simulink model "ranqilunji"  (R2014a)
settings: Solver=ode45  StartTime=0.0  StopTime=10.0  RelTol=1e-3
settings Model: Creator=Administrator  LastModifiedBy=Administrator

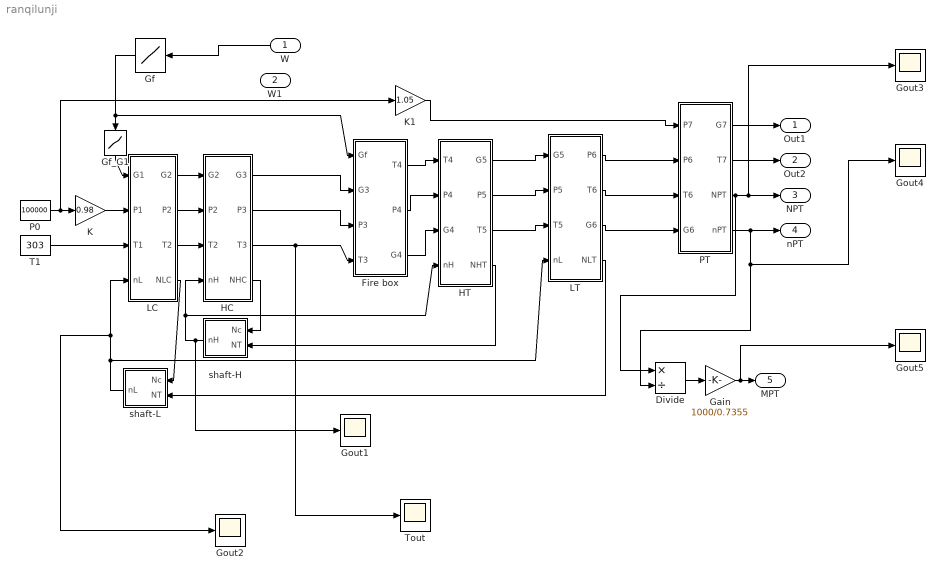
== system ranqilunji ==
  W : Inport
  W1 : Inport  Port=2
  Divide : Product  Inputs=*/
  Fire box : Subsystem
  Gain : Gain  Gain=1000/0.7355
  Gf : Lookup  InputValues=[0,0.03,0.07,0.09,0.11,0.13,0.17,0.2,0.23,0.26,0.28,0.3,0.32,0.34,0.35,0.38,0.4,0.42,0.44,0.47,0.49,0.5,0.52,0.54,0.55,0.59,0.61,0.64,0.66,0.68,0.7,0.72,0.74,0.77,0.81,0.83,0.85,0.88,0.93,0.95,0.97,1]  Table=[0.172,0.236,0.331,0.331,0.366,0.411,0.488,0.536,0.582,0.605,0.644,0.682,0.698,0.728,0.727,0.783,0.783,0.813,0.857,0.886,0.935,0.949,0.95,0.975,0.999,1.022,1.069,1.149,1.153,1.184,1.206,1.233,1.256,1.271,1.325,1.383,1.383,1.439,1.481,1.504,1.52,1.574]
  Gf_G1 : Lookup  InputValues=[0.172,0.236,0.331,0.366,0.411,0.488,0.536,0.582,0.605,0.644,0.682,0.698,0.727,0.728,0.783,0.813,0.857,0.886,0.935,0.949,0.95,0.975,0.999,1.022,1.069,1.149,1.153,1.184,1.206,1.233,1.256,1.271,1.325,1.383,1.439,1.481,1.504,1.52,1.574]  Table="[20.01, 25.93, 38.77,  43.65, 45.94, 51.85, 54.70, 56.85, 59.03, 61.91, 60.44, 61.58, 62.93, 63.04, 65.71,   67.00, 69.52, 70.63, 73.19, 73.46, 73.44, 73.83, 75.62, 76.39, 78.27, 81.17, 81.50, 82.44, 83.44, 84.31, 85.30, 86.17, 87.93, 89.72, 91.51, 93.65, 94.63, 94.92, 97.64]"
  Gout{1..5} (5 alike) : Scope
      Gout1 settings: TimeRange=10
      Gout2 settings: TimeRange=10  SaveName=ScopeData3
      Gout3 settings: TimeRange=10  SaveName=ScopeData21
      Gout4 settings: TimeRange=10  SaveName=ScopeData2
      Gout5 settings: TimeRange=10  SaveName=ScopeData5
  HC : Subsystem
  HT : Subsystem
  K : Gain  Gain=0.98
  K1 : Gain  Gain=1.05
  LC : Subsystem
  LT : Subsystem
  P0 : Constant  Value=100000
  PT : Subsystem
  T1 : Constant  Value=303
  Tout : Scope
      settings: TimeRange=200  YMin=740  YMax=790
  shaft-H : Subsystem  mask(rotor module){J=30}
      mask prompts: J "J moment of inertia(Nm)"
      mask help: (pi^2*J*n/900)*(dn/dt)=NT-Nc
  shaft-L : Subsystem  mask(rotor module){J=15}
      mask prompts: J "J moment of inertia(Nm)"
      mask help: (pi^2*J*n/900)*(dn/dt)=NT-Nc
  Out1 : Outport
  Out2 : Outport  Port=2
  NPT : Outport  Port=3
  nPT : Outport  Port=4
  MPT : Outport  Port=5
  wires:
  T1/1 -> LC/3(T1)
  K/1 -> LC/2(P1)
  LC/1(G2) -> HC/1(G2)
  LC/2(P2) -> HC/2(P2)
  LC/3(T2) -> HC/3(T2)
  HC/1(G3) -> Fire box/2(G3)
  HC/2(P3) -> Fire box/3(P3)
  HC/3(T3) -> Fire box/4(T3), Tout/1
  HC/4(NHC) -> shaft-H/1(Nc)
  HT/4(NHT) -> shaft-H/2(NT)
  shaft-H/1(nH) -> HT/4(nH), HC/4(nH), Gout1/1
  LC/4(NLC) -> shaft-L/1(Nc)
  LT/4(NLT) -> shaft-L/2(NT)
  Gf/1 -> Gf_G1/1, Fire box/1(Gf)
  Gf_G1/1 -> LC/1(G1)
  Fire box/3(G4) -> HT/3(G4)
  Fire box/2(P4) -> HT/2(P4)
  HT/3(T5) -> LT/3(T5)
  HT/2(P5) -> LT/2(P5)
  HT/1(G5) -> LT/1(G5)
  LT/3(G6) -> PT/4(G6)
  LT/2(T6) -> PT/3(T6)
  shaft-L/1(nL) -> LT/4(nL), LC/4(nL), Gout2/1
  LT/1(P6) -> PT/2(P6)
  P0/1 -> K/1, K1/1
  Fire box/1(T4) -> HT/1(T4)
  K1/1 -> PT/1(P7)
  W/1 -> Gf/1
  PT/1(G7) -> Out1/1
  PT/2(T7) -> Out2/1
  PT/3(NPT) -> Gout3/1, NPT/1, Divide/1
  PT/4(nPT) -> nPT/1, Gout4/1, Divide/2
  Gain/1 -> Gout5/1, MPT/1
  Divide/1 -> Gain/1

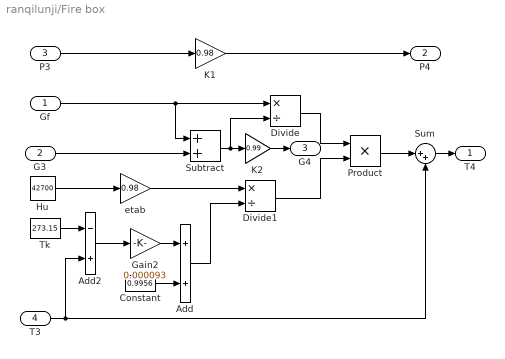
== system ranqilunji/Fire box ==
  Gf : Inport
  G3 : Inport  Port=2
  P3 : Inport  Port=3
  T3 : Inport  Port=4
  Add : Sum
  Add2 : Sum  Inputs=-+
  Constant : Constant  Value=0.9956
  Divide : Product  Inputs=*/
  Divide1 : Product  Inputs=*/
  Gain2 : Gain  Gain=0.000093
  Hu : Constant  Value=42700
  K1 : Gain  Gain=0.98
  K2 : Gain  Gain=0.99
  Product : Product  RndMeth=Zero
  Subtract : Sum
  Sum : Sum  Inputs=|++
  Tk : Constant  Value=273.15
  etab : Gain  Gain=0.98
  T4 : Outport
  P4 : Outport  Port=2
  G4 : Outport  Port=3
  wires:
  Gf/1 -> Divide/1, Subtract/1
  Divide/1 -> Product/1
  G3/1 -> Subtract/2
  Subtract/1 -> Divide/2, K2/1
  Hu/1 -> etab/1
  etab/1 -> Divide1/1
  Divide1/1 -> Product/2
  Product/1 -> Sum/1
  Sum/1 -> T4/1
  T3/1 -> Add2/2, Sum/2
  P3/1 -> K1/1
  K1/1 -> P4/1
  Constant/1 -> Add/2
  Gain2/1 -> Add/1
  Tk/1 -> Add2/1
  Add2/1 -> Gain2/1
  Add/1 -> Divide1/2
  K2/1 -> G4/1

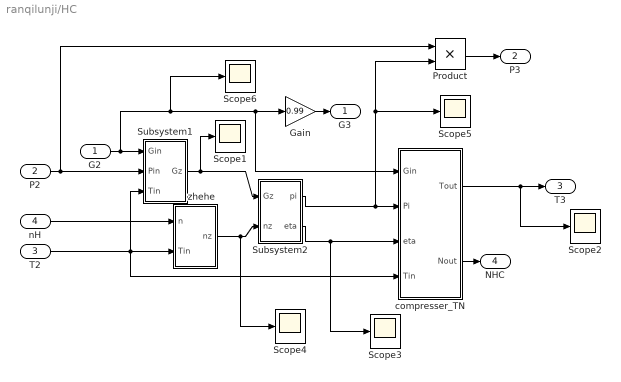
== system ranqilunji/HC ==
  G2 : Inport
  P2 : Inport  Port=2
  T2 : Inport  Port=3
  nH : Inport  Port=4
  Gain : Gain  Gain=0.99
  Product : Product  RndMeth=Zero
  Scope{1..6} (6 alike) : Scope
      Scope1 settings: YMin=2829.54  YMax=3127.38  SaveName=ScopeData16
      Scope2 settings: YMin=2829.54  YMax=3127.38  SaveName=ScopeData29
      Scope3 settings: YMin=2829.54  YMax=3127.38  SaveName=ScopeData24
      Scope4 settings: YMin=2829.54  YMax=3127.38  SaveName=ScopeData31
      Scope5 settings: YMin=2829.54  YMax=3127.38  SaveName=ScopeData10
      Scope6 settings: YMin=2829.54  YMax=3127.38  SaveName=ScopeData15
  Subsystem1 : Subsystem
  Subsystem2 : Subsystem
  compresser_TN : Subsystem  mask(Compressor_Tout Nout module){}
  zhehe : Subsystem
  G3 : Outport
  P3 : Outport  Port=2
  T3 : Outport  Port=3
  NHC : Outport  Port=4
  wires:
  zhehe/1(nz) -> Scope4/1, Subsystem2/2(nz)
  Subsystem2/1(pi) -> compresser_TN/2(Pi), Product/2, Scope5/1
  Subsystem2/2(eta) -> compresser_TN/3(eta), Scope3/1
  T2/1 -> zhehe/2(Tin), compresser_TN/4(Tin), Subsystem1/3(Tin)
  nH/1 -> zhehe/1(n)
  Gain/1 -> G3/1
  compresser_TN/1(Tout) -> T3/1, Scope2/1
  compresser_TN/2(Nout) -> NHC/1
  Subsystem1/1(Gz) -> Scope1/1, Subsystem2/1(Gz)
  G2/1 -> Subsystem1/1(Gin), Gain/1, compresser_TN/1(Gin), Scope6/1
  P2/1 -> Subsystem1/2(Pin), Product/1
  Product/1 -> P3/1

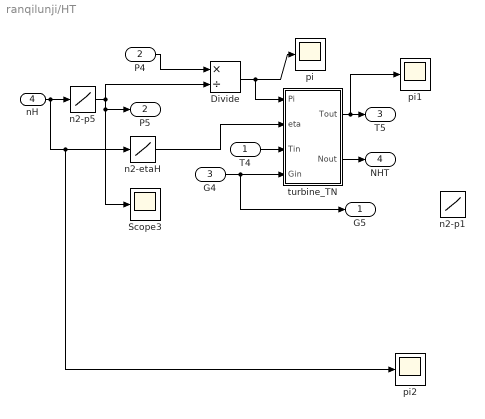
== system ranqilunji/HT ==
  T4 : Inport
  P4 : Inport  Port=2
  G4 : Inport  Port=3
  nH : Inport  Port=4
  Divide : Product  Inputs=*/
  Scope3 : Scope
      settings: TimeRange=100  YMin=5000  YMax=25000  SaveName=ScopeData34
  n2-etaH : Lookup  InputValues=[6000 6300 6500 6800 7000 7150 7300 7500 7800]  Table=[0.81 0.83 0.85 0.87 0.88 0.87 0.86 0.855 0.85]
  n2-p1 : Lookup  InputValues=[6000 6503 6995 7498 8002 8505 8997 9500]  Table=[139400 150700 186000 246700 332500 443400 575800 736100]
  n2-p5 : Lookup  InputValues=[5832,7212,7282,7644,7752,7853,8033,8092 8211 8392 8430 8452 8670 8767 8960 8999 9073]  Table=[154000,269000,296000,361000,391000,419000,476000,494000 534000 596000 609000 616000 684000 719000 806000 814000 831000]
  pi : Scope
      settings: TimeRange=100  YMin=2829.54  YMax=3127.38  SaveName=ScopeData17
  pi1 : Scope
      settings: TimeRange=100  YMin=2829.54  YMax=3127.38  SaveName=ScopeData7
  pi2 : Scope
      settings: TimeRange=100  YMin=2829.54  YMax=3127.38  SaveName=ScopeData35
  turbine_TN : Subsystem  mask(Turbine_Tout Nout module){}
  G5 : Outport
  P5 : Outport  Port=2
  T5 : Outport  Port=3
  NHT : Outport  Port=4
  wires:
  n2-etaH/1 -> turbine_TN/2(eta)
  P4/1 -> Divide/1
  nH/1 -> pi2/1, n2-etaH/1, n2-p5/1
  turbine_TN/1(Tout) -> T5/1, pi1/1
  T4/1 -> turbine_TN/3(Tin)
  turbine_TN/2(Nout) -> NHT/1
  G4/1 -> turbine_TN/4(Gin), G5/1
  Divide/1 -> turbine_TN/1(Pi), pi/1
  n2-p5/1 -> Divide/2, P5/1, Scope3/1

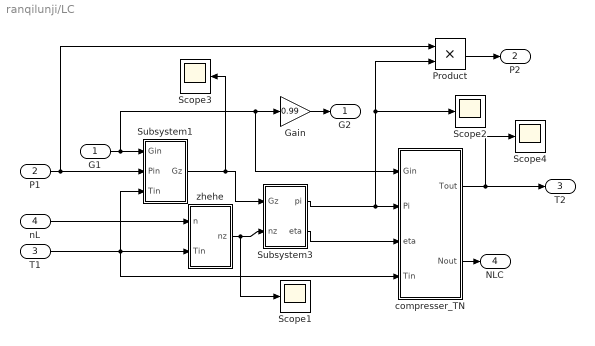
== system ranqilunji/LC ==
  G1 : Inport
  P1 : Inport  Port=2
  T1 : Inport  Port=3
  nL : Inport  Port=4
  Gain : Gain  Gain=0.99
  Product : Product  RndMeth=Zero
  Scope{1..4} (4 alike) : Scope
      Scope1 settings: YMin=2829.54  YMax=3127.38  SaveName=ScopeData14
      Scope2 settings: YMin=2829.54  YMax=3127.38  SaveName=ScopeData9
      Scope3 settings: YMin=2829.54  YMax=3127.38  SaveName=ScopeData30
      Scope4 settings: TimeRange=80  YMin=5000  YMax=30000  SaveName=ScopeData32
  Subsystem1 : Subsystem
  Subsystem3 : Subsystem
  compresser_TN : Subsystem  mask(Compressor_Tout Nout module){}
  zhehe : Subsystem
  G2 : Outport
  P2 : Outport  Port=2
  T2 : Outport  Port=3
  NLC : Outport  Port=4
  wires:
  zhehe/1(nz) -> Scope1/1, Subsystem3/2(nz)
  Subsystem3/1(pi) -> compresser_TN/2(Pi), Product/2, Scope2/1
  Subsystem3/2(eta) -> compresser_TN/3(eta)
  T1/1 -> zhehe/2(Tin), compresser_TN/4(Tin), Subsystem1/3(Tin)
  nL/1 -> zhehe/1(n)
  Gain/1 -> G2/1
  compresser_TN/1(Tout) -> T2/1, Scope4/1
  compresser_TN/2(Nout) -> NLC/1
  Subsystem1/1(Gz) -> Scope3/1, Subsystem3/1(Gz)
  G1/1 -> Subsystem1/1(Gin), Gain/1, compresser_TN/1(Gin)
  P1/1 -> Subsystem1/2(Pin), Product/1
  Product/1 -> P2/1

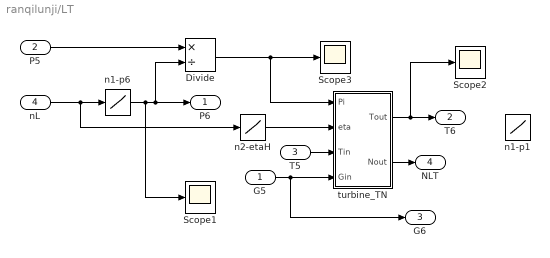
== system ranqilunji/LT ==
  G5 : Inport
  P5 : Inport  Port=2
  T5 : Inport  Port=3
  nL : Inport  Port=4
  Divide : Product  Inputs=*/
  Scope1 : Scope
      settings: TimeRange=100  YMin=5000  YMax=25000  SaveName=ScopeData28
  Scope2 : Scope
      settings: TimeRange=100  YMin=5000  YMax=25000  SaveName=ScopeData4
  Scope3 : Scope
      settings: TimeRange=100  YMin=5000  YMax=25000  SaveName=ScopeData20
  n1-p1 : Lookup  InputValues="[2849,4651,4850,5410,5586,5742,6024,6092,6102,6211,6385,6425 6435 6609 6698  6732 7015  7080 7185 ]"  Table="[101000,131000,141000,161000,171000,181000,201000,201000,211000,221000,241000,251000 251000 281000 291000  301000 321000  331000 341000]"
  n1-p6 : Lookup  InputValues=[2849,4651,4850,5410,5586,5742,6024,6092,6102,6211,6385,6425,6435,6609,6698,6732,7015,7080,7185]  Table=[113000,150000,157000,180000,190000,201000,221000,229000,229500,242000,267000,272000,277000,306000,321000,322000,354000,360000,371000]
  n2-etaH : Lookup  InputValues=[4300 5000 5500 6000 6500 7000 7500 8000 9000 9500]  Table=[0.82 0.83 0.835 0.84 0.85 0.86 0.875 0.87 0.865 0.86]
  turbine_TN : Subsystem  mask(Turbine_Tout Nout module){}
  P6 : Outport
  T6 : Outport  Port=2
  G6 : Outport  Port=3
  NLT : Outport  Port=4
  wires:
  n2-etaH/1 -> turbine_TN/2(eta)
  P5/1 -> Divide/1
  nL/1 -> n2-etaH/1, n1-p6/1
  turbine_TN/1(Tout) -> T6/1, Scope2/1
  T5/1 -> turbine_TN/3(Tin)
  turbine_TN/2(Nout) -> NLT/1
  G5/1 -> turbine_TN/4(Gin), G6/1
  n1-p6/1 -> Divide/2, P6/1, Scope1/1
  Divide/1 -> turbine_TN/1(Pi), Scope3/1

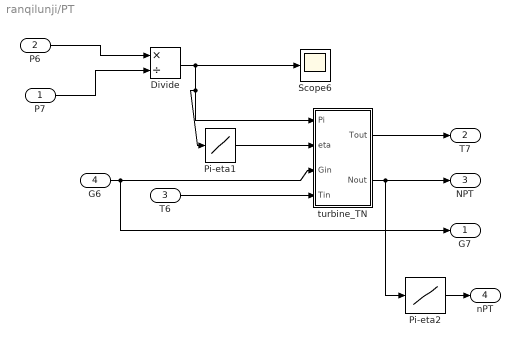
== system ranqilunji/PT ==
  P7 : Inport
  P6 : Inport  Port=2
  T6 : Inport  Port=3
  G6 : Inport  Port=4
  Divide : Product  Inputs=*/
  Pi-eta1 : Lookup  InputValues=[1,1.11 1.41 1.51 1.81 2.0 2.21 2.41 2.61 2.81]  Table=[0.825,0.83 0.85 0.86 0.88 0.90 0.905 0.91 0.905 0.9]
  Pi-eta2 : Lookup  InputValues=[307,625,1634,2141,2611,3121,4030,4941,5687,6256,6755,7309,7716,8175,8374,9153,9719,10196,10702,11284,11832,12033,12512,13051,13298,14334,14778,15580,16003,16531,16669,17381,17948,18600,19648,20212,20613,21462,22525,23139,23520,24372]  Table=[878,1243,1778,1749,1547,1574,1765,1930,2049,2045,2069,2150,2158,2185,2214,2272,2274,2209,2231,2240,2252,2500,2569,2649,2574,2650,2617,2639,2697,2653,2702,2785,2901,2979,3042,2919,2951,3108,3089,3056,3065,3142]
  Scope6 : Scope
      settings: YMin=2829.54  YMax=3127.38  SaveName=ScopeData22
  turbine_TN : Subsystem  mask(Turbine_Tout Nout module){}
  G7 : Outport
  T7 : Outport  Port=2
  NPT : Outport  Port=3
  nPT : Outport  Port=4
  wires:
  turbine_TN/1(Tout) -> T7/1
  turbine_TN/2(Nout) -> NPT/1, Pi-eta2/1
  G6/1 -> turbine_TN/3(Gin), G7/1
  Divide/1 -> Scope6/1, turbine_TN/1(Pi), Pi-eta1/1
  T6/1 -> turbine_TN/4(Tin)
  Pi-eta1/1 -> turbine_TN/2(eta)
  P6/1 -> Divide/1
  P7/1 -> Divide/2
  Pi-eta2/1 -> nPT/1

== system ranqilunji/shaft-H ==
  Nc : Inport
  NT : Inport  Port=2
  Add : Sum  Inputs=-+
  Divide : Product  Inputs=3
  Fcn : Fcn  Expr=1/u
  Fcn1 : Fcn  Expr=1/u
  Gain : Gain  Gain=15/(pi*pi)
  Gain3 : Gain  Gain=60
  Integrator : Integrator  InitialCondition=143.58
  J : Constant  Value=J
  nH : Outport
  wires:
  Nc/1 -> Add/1
  NT/1 -> Add/2
  Divide/1 -> Integrator/1
  Integrator/1 -> Fcn1/1, Gain3/1
  Add/1 -> Divide/1
  J/1 -> Fcn/1
  Gain/1 -> Divide/2
  Fcn/1 -> Gain/1
  Fcn1/1 -> Divide/3
  Gain3/1 -> nH/1

== system ranqilunji/shaft-L ==
  Nc : Inport
  NT : Inport  Port=2
  Add : Sum  Inputs=-+
  Divide : Product  Inputs=3
  Fcn : Fcn  Expr=1/u
  Fcn1 : Fcn  Expr=1/u
  Gain : Gain  Gain=15/(pi*pi)
  Gain2 : Gain  Gain=60
  Integrator : Integrator  InitialCondition=105.9
  J : Constant  Value=J
  nL : Outport
  wires:
  Nc/1 -> Add/1
  NT/1 -> Add/2
  Divide/1 -> Integrator/1
  Integrator/1 -> Fcn1/1, Gain2/1
  Add/1 -> Divide/1
  J/1 -> Fcn/1
  Gain/1 -> Divide/2
  Fcn/1 -> Gain/1
  Fcn1/1 -> Divide/3
  Gain2/1 -> nL/1

== system ranqilunji/HC/Subsystem1 ==
  Gin : Inport
  Pin : Inport  Port=2
  Tin : Inport  Port=3
  Divide : Product  Inputs=*/
  Divide1 : Product  Inputs=*/
  Divide2 : Product  Inputs=*/
  Fcn : Fcn  Expr=sqrt(u)
  P0 : Constant  Value=100000
  Product : Product  RndMeth=Zero
  T0 : Constant  Value=288
  Gz : Outport
  wires:
  Tin/1 -> Divide/1
  T0/1 -> Divide/2
  Divide/1 -> Fcn/1
  Pin/1 -> Divide1/1
  P0/1 -> Divide1/2
  Gin/1 -> Divide2/1
  Divide1/1 -> Divide2/2
  Fcn/1 -> Product/1
  Divide2/1 -> Product/2
  Product/1 -> Gz/1

== system ranqilunji/HC/Subsystem2 ==
  Gz : Inport
  nz : Inport  Port=2
  Lookup Table (2-D) : Lookup2D  RowIndex=[6000 6300 6500 6800 7000 7300 7500 7800]  ColumnIndex=[12:0.2:29]  Table=|
      | [2.4803 2.5510 2.6217 2.6924 2.7630 2.8337 2.9044 2.9751 3.0172 2.9863 2.9541 2.9206 2.8860 2.8500 2.8129 2.7745 2.7349 2.6940 2.6519 2.6085 2.5640 2.5181 2.4711 2.4906 2.5237 2.5573 2.5913 2.6257 2.6605 2.6958 2.7314 2.7675 2.8040 2.8409 2.8783 2.9161 2.9543 2.9929 3.0319 3.0714 3.1112 3.1515 3.1923 3.2334 3.2750 3.3169 3.3593 3.4022 3.4454 3.4891 3.5332 3.5777 3.6226 3.6679 3.7137 3.7599 3.8065 3.8535 3.9010 3.9488 3.9971 4.0307 4.0450 4.0645  4.0889 4.0613 4.0669 4.0759 4.0882 4.1107 4.1332 4.1561 4.2095 4.2632 4.3174 4.3720 4.4271 4.4825 4.5384 4.5947 4.6514 4.7085 4.7660 4.8240 4.8824 5.0412;
      | 2.4803 2.5510 2.6217 2.6924 2.7630 2.8337 2.9044 2.9751 3.0457 3.1164 3.1871 3.2578 3.3284 3.3991 3.5124 3.4922 3.4694 3.4440 3.4159 3.3853 3.3520 3.3161 3.2775 3.2364 3.1926 3.1462 3.0972 3.0456 2.9914 2.9345 2.8750 2.8129 2.8040 2.8409 2.8783 2.9161 2.9543 2.9929 3.0319 3.0714 3.1112 3.1515 3.1923 3.2334 3.2750 3.3169 3.3593 3.4022 3.4454 3.4891 3.5332 3.5777 3.6226 3.6679 3.7137 3.7599 3.8065 3.8535 3.9010 3.9488 3.9971 4.0307 4.0450 4.0645  4.0889 4.0613 4.0669 4.0759 4.0882 4.1107 4.1332 4.1561 4.2095 4.2632 4.3174 4.3720 4.4271 4.4825 4.5384 4.5947 4.6514 4.7085 4.7660 4.8240 4.8824 5.0412;
      | 2.4803 2.5510 2.6217 2.6924 2.7630 2.8337 2.9044 2.9751 3.0457 3.1164 3.1871 3.2578 3.3284 3.3991 3.4698 3.5405 3.6111 3.6818 3.7525 3.8394 3.8358 3.8266 3.8119 3.7916 3.7659 3.7345 3.6977 3.6553 3.6073 3.5539 3.4948 3.4303 3.3602 3.2845 3.2034 3.1167 3.0244 2.9929 3.0319 3.0714 3.1112 3.1515 3.1923 3.2334 3.2750 3.3169 3.3593 3.4022 3.4454 3.4891 3.5332 3.5777 3.6226 3.6679 3.7137 3.7599 3.8065 3.8535 3.9010 3.9488 3.9971 4.0307 4.0450 4.0645  4.0889 4.0613 4.0669 4.0759 4.0882 4.1107 4.1332 4.1561 4.2095 4.2632 4.3174 4.3720 4.4271 4.4825 4.5384 4.5947 4.6514 4.7085 4.7660 4.8240 4.8824 5.0412;
      | 2.4803 2.5510 2.6217 2.6924 2.7630 2.8337 2.9044 2.9751 3.0457 3.1164 3.1871 3.2578 3.3284 3.3991 3.4698 3.5405 3.6111 3.6818 3.7525 3.8231 3.8938 3.9645 4.0352 4.1058 4.1765 4.2472 4.3179 4.4049 4.4021 4.3892 4.3664 4.3334 4.2904 4.2374 4.1744 4.1012 4.0181 3.9249 3.8216 3.7083 3.5850 3.4516 3.3082 3.2334 3.2750 3.3169 3.3593 3.4022 3.4454 3.4891 3.5332 3.5777 3.6226 3.6679 3.7137 3.7599 3.8065 3.8535 3.9010 3.9488 3.9971 4.0307 4.0450 4.0645  4.0889 4.0613 4.0669 4.0759 4.0882 4.1107 4.1332 4.1561 4.2095 4.2632 4.3174 4.3720 4.4271 4.4825 4.5384 4.5947 4.6514 4.7085 4.7660 4.8240 4.8824 5.0412;
      | 2.4803 2.5510 2.6217 2.6924 2.7630 2.8337 2.9044 2.9751 3.0457 3.1164 3.1871 3.2578 3.3284 3.3991 3.4698 3.5405 3.6111 3.6818 3.7525 3.8231 3.8938 3.9645 4.0352 4.1058 4.1765 4.2472 4.3179 4.3885 4.4592 4.5299 4.6006 4.6379 4.6228 4.5996 4.5680 4.5283 4.4803 4.4241 4.3596 4.2869 4.2060 4.1168 4.0195 3.9138 3.8000 3.6779 3.5476 3.4090 3.4054 3.4591 3.5000 3.5277 3.5426 3.5679 3.5837 3.5999 3.8065 3.8535 3.9010 3.9488 3.9971 4.0307 4.0450 4.0645  4.0889 4.0613 4.0669 4.0759 4.0882 4.1107 4.1332 4.1561 4.2095 4.2632 4.3174 4.3720 4.4271 4.4825 4.5384 4.5947 4.6514 4.7085 4.7660 4.8240 4.8824 5.0412;
      | 2.4803 2.5510 2.6217 2.6924 2.7630 2.8337 2.9044 2.9751 3.0457 3.1164 3.1871 3.2578 3.3284 3.3991 3.4698 3.5405 3.6111 3.6818 3.7525 3.8231 3.8938 3.9645 4.0352 4.1058 4.1765 4.2472 4.3179 4.3885 4.4592 4.5299 4.6006 4.6712 4.7419 4.8126 4.8833 4.9539 5.0246 5.0953 5.1660 5.2000 5.1000 5.0000 4.9700 4.9000 4.8200 4.6810 4.6468 4.6015 4.5451 4.4775 4.3988 4.3090 4.2081 4.0961 3.9729 3.8386 3.8065 3.8535 3.9010 3.9488 3.9971 4.0307 4.0450 4.0645  4.0889 4.0613 4.0669 4.0759 4.0882 4.1107 4.1332 4.1561 4.2095 4.2632 4.3174 4.3720 4.4271 4.4825 4.5384 4.5947 4.6514 4.7085 4.7660 4.8240 4.8824 5.0412;
      | 2.4803 2.5510 2.6217 2.6924 2.7630 2.8337 2.9044 2.9751 3.0457 3.1164 3.1871 3.2578 3.3284 3.3991 3.4698 3.5405 3.6111 3.6818 3.7525 3.8231 3.8938 3.9645 4.0352 4.1058 4.1765 4.2472 4.3179 4.3885 4.4592 4.5299 4.6006 4.6712 4.7419 4.8126 4.8833 4.9539 5.0246 5.0953 5.1660 5.2366 5.3073 5.3780 5.4486 5.5193 5.5000 5.4500 5.4000 5.3500 5.3000 5.2500 5.2036 5.1763 5.1322 5.0715 4.9940 4.8998 4.7889 4.6613 4.5169 4.3559 4.0182 4.0307 4.0450 4.0645 4.0889 4.0613 4.0669 4.0759 4.0882 4.1107 4.1332 4.1561 4.2095 4.2632 4.3174 4.3720 4.4271 4.4825 4.5384 4.5947 4.6514 4.7085 4.7660 4.8240 4.8824 5.0412; 
      | 2.4803 2.5510 2.6217 2.6924 2.7630 2.8337 2.9044 2.9751 3.0457 3.1164 3.1871 3.2578 3.3284 3.3991 3.4698 3.5405 3.6111 3.6818 3.7525 3.8231 3.8938 3.9645 4.0352 4.1058 4.1765 4.2472 4.3179 4.3885 4.4592 4.5299 4.6006 4.6712 4.7419 4.8126 4.8833 4.9539 5.0246 5.0953 5.1660 5.2366 5.3073 5.3780 5.4486 5.5193 5.5900 5.6607 5.7313 5.8020 5.8727 5.9434 6.0140 6.0847 6.1554 6.2261 6.2967 6.3674 6.4381 6.5088 5.5861 5.3841 5.1514 4.8878 4.5936 4.0685 4.0889 4.0613 4.0669 4.0759 4.0882 4.1107 4.1332 4.1561 4.2095 4.2632 4.3174 4.3720 4.4271 4.4825 4.5384 4.5947 4.6514 4.7085 4.7660 4.8240 4.8824 5.0412;]
  Lookup Table (2-D)1 : Lookup2D  RowIndex=[6000 6300 6500 6800 7000 7300 7500 7800]  ColumnIndex=[12:0.2:29]  Table=|
      | [0.8450 0.8455 0.8460 0.8465 0.8470 0.8480 0.8490 0.8495 0.8500 0.8510 0.8520 0.8530 0.8540 0.8540 0.8540 0.8525 0.8510 0.8500 0.8490 0.8480 0.8470 0.8460 0.8450 0.8455 0.8460 0.8460 0.8460 0.8470 0.8480 0.8480 0.8480 0.8480 0.8480 0.8485 0.8490 0.8490 0.8490 0.8490 0.8490 0.8490 0.8490 0.8490 0.8490 0.8490 0.8490 0.8490 0.8490 0.8490 0.8490 0.8495 0.8500 0.8500 0.8500 0.8500 0.8500 0.8500 0.8500 0.8495 0.8490 0.8495 0.8500 0.8490 0.8480 0.8480 0.8480 0.8475 0.8470 0.8465 0.8460 0.8455 0.8450 0.8445 0.8440 0.8435 0.8430 0.8425 0.8420 0.8415 0.8410 0.8405 0.8400 0.8395 0.8390 0.8385 0.8380 0.8375;
      | 0.8450 0.8455 0.8460 0.8465 0.8470 0.8480 0.8490 0.8495 0.8500 0.8505 0.8510 0.8515 0.8520 0.8520 0.8520 0.8556 0.8597 0.8631 0.8658 0.8678 0.8691 0.8697 0.8696 0.8688 0.8672 0.8650 0.8621 0.8585 0.8542 0.8492 0.8435 0.8371 0.8480 0.8485 0.8490 0.8490 0.8490 0.8490 0.8490 0.8490 0.8490 0.8490 0.8490 0.8490 0.8490 0.8490 0.8490 0.8490 0.8490 0.8495 0.8500 0.8500 0.8500 0.8500 0.8500 0.8500 0.8500 0.8495 0.8490 0.8495 0.8500 0.8490 0.8480 0.8480 0.8480 0.8475 0.8470 0.8465 0.8460 0.8455 0.8450 0.8445 0.8440 0.8435 0.8430 0.8425 0.8420 0.8415 0.8410 0.8405 0.8400 0.8395 0.8390 0.8385 0.8380 0.8375;
      | 0.8450 0.8455 0.8460 0.8465 0.8470 0.8480 0.8490 0.8495 0.8500 0.8505 0.8510 0.8515 0.8520 0.8520 0.8520 0.8525 0.8530 0.8530 0.8530 0.8611 0.8688 0.8754 0.8809 0.8854 0.8888 0.8910 0.8922 0.8923 0.8914 0.8893 0.8861 0.8819 0.8766 0.8702 0.8627 0.8541 0.8444 0.8490 0.8490 0.8490 0.8490 0.8490 0.8490 0.8490 0.8490 0.8490 0.8490 0.8490 0.8490 0.8495 0.8500 0.8500 0.8500 0.8500 0.8500 0.8500 0.8500 0.8495 0.8490 0.8495 0.8500 0.8490 0.8480 0.8480 0.8480 0.8475 0.8470 0.8465 0.8460 0.8455 0.8450 0.8445 0.8440 0.8435 0.8430 0.8425 0.8420 0.8415 0.8410 0.8405 0.8400 0.8395 0.8390 0.8385 0.8380 0.8375;
      | 0.8450 0.8455 0.8460 0.8465 0.8470 0.8480 0.8490 0.8495 0.8500 0.8505 0.8510 0.8515 0.8520 0.8520 0.8520 0.8525 0.8530 0.8530 0.8530 0.8540 0.8550 0.8565 0.8580 0.8600 0.8620 0.8630 0.8640 0.8669 0.8710 0.8830 0.8930 0.9010 0.9070 0.9110 0.9129 0.9129 0.9108 0.9067 0.9006 0.8925 0.8824 0.8703 0.8561 0.8490 0.8490 0.8490 0.8490 0.8490 0.8490 0.8495 0.8500 0.8500 0.8500 0.8500 0.8500 0.8500 0.8500 0.8495 0.8490 0.8495 0.8500 0.8490 0.8480 0.8480 0.8480 0.8475 0.8470 0.8465 0.8460 0.8455 0.8450 0.8445 0.8440 0.8435 0.8430 0.8425 0.8420 0.8415 0.8410 0.8405 0.8400 0.8395 0.8390 0.8385 0.8380 0.8375;
      | 0.8450 0.8455 0.8460 0.8465 0.8470 0.8480 0.8490 0.8495 0.8500 0.8505 0.8510 0.8515 0.8520 0.8520 0.8520 0.8525 0.8530 0.8530 0.8530 0.8540 0.8550 0.8565 0.8580 0.8600 0.8620 0.8630 0.8640 0.8505 0.8500 0.8500 0.8500 0.8499 0.8618 0.8720 0.8808 0.8879 0.8935 0.8975 0.8999 0.9008 0.9001 0.8978 0.8940 0.8886 0.8816 0.8731 0.8630 0.8513 0.8490 0.8495 0.8500 0.8500 0.8500 0.8500 0.8500 0.8500 0.8500 0.8495 0.8490 0.8495 0.8500 0.8490 0.8480 0.8480 0.8480 0.8475 0.8470 0.8465 0.8460 0.8455 0.8450 0.8445 0.8440 0.8435 0.8430 0.8425 0.8420 0.8415 0.8410 0.8405 0.8400 0.8395 0.8390 0.8385 0.8380 0.8375;
      | 0.8450 0.8455 0.8460 0.8465 0.8470 0.8480 0.8490 0.8495 0.8500 0.8505 0.8510 0.8515 0.8520 0.8520 0.8520 0.8525 0.8530 0.8530 0.8530 0.8540 0.8550 0.8565 0.8580 0.8600 0.8620 0.8630 0.8640 0.8505 0.8500 0.8500 0.8500 0.8495 0.8490 0.8485 0.8480 0.8475 0.8470 0.8470 0.8470 0.8586 0.8661 0.8726 0.8781 0.8825 0.8860 0.8884 0.8897 0.8901 0.8894 0.8878 0.8851 0.8813 0.8766 0.8708 0.8640 0.8562 0.8500 0.8495 0.8490 0.8495 0.8500 0.8490 0.8480 0.8480 0.8480 0.8475 0.8470 0.8465 0.8460 0.8455 0.8450 0.8445 0.8440 0.8435 0.8430 0.8425 0.8420 0.8415 0.8410 0.8405 0.8400 0.8395 0.8390 0.8385 0.8380 0.8375;
      | 0.8450 0.8455 0.8460 0.8465 0.8470 0.8480 0.8490 0.8495 0.8500 0.8505 0.8510 0.8515 0.8520 0.8520 0.8520 0.8525 0.8530 0.8530 0.8530 0.8540 0.8550 0.8565 0.8580 0.8600 0.8620 0.8630 0.8640 0.8505 0.8500 0.8500 0.8500 0.8495 0.8490 0.8485 0.8480 0.8475 0.8470 0.8470 0.8470 0.8465 0.8460 0.8455 0.8450 0.8450 0.8450 0.8460 0.8456 0.8496 0.8528 0.8554 0.8572 0.8582 0.8585 0.8581 0.8569 0.8550 0.8523 0.8500 0.8500 0.8495 0.8495 0.8490 0.8480 0.8480 0.8480 0.8475 0.8470 0.8465 0.8460 0.8455 0.8450 0.8445 0.8440 0.8435 0.8430 0.8425 0.8420 0.8415 0.8410 0.8405 0.8400 0.8395 0.8390 0.8385 0.8380 0.8375;
      | 0.8450 0.8455 0.8460 0.8465 0.8470 0.8480 0.8490 0.8495 0.8500 0.8505 0.8510 0.8515 0.8520 0.8520 0.8520 0.8525 0.8530 0.8530 0.8530 0.8540 0.8550 0.8565 0.8580 0.8600 0.8620 0.8630 0.8640 0.8505 0.8500 0.8500 0.8500 0.8495 0.8490 0.8485 0.8480 0.8475 0.8470 0.8470 0.8470 0.8465 0.8460 0.8455 0.8450 0.8450 0.8450 0.8445 0.8440 0.8445 0.8450 0.8445 0.8440 0.8425 0.8400 0.8415 0.8430 0.8455 0.8480 0.8510 0.8550 0.8600 0.8650 0.8650 0.8650 0.8650 0.8480 0.8475 0.8470 0.8465 0.8460 0.8455 0.8450 0.8445 0.8440 0.8435 0.8430 0.8425 0.8420 0.8415 0.8410 0.8405 0.8400 0.8395 0.8390 0.8385 0.8380 0.8375;]
  pi : Outport
  eta : Outport  Port=2
  wires:
  nz/1 -> Lookup Table (2-D)/1, Lookup Table (2-D)1/1
  Gz/1 -> Lookup Table (2-D)1/2, Lookup Table (2-D)/2
  Lookup Table (2-D)/1 -> pi/1
  Lookup Table (2-D)1/1 -> eta/1

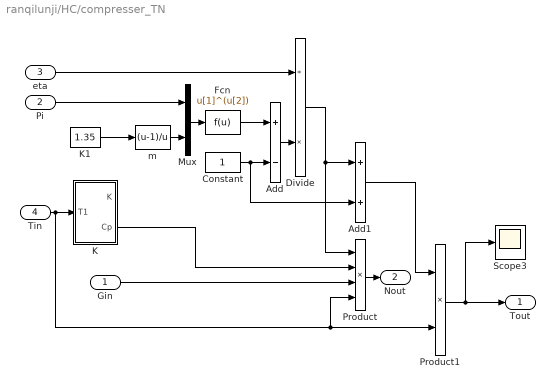
== system ranqilunji/HC/compresser_TN ==
  Gin : Inport
  Pi : Inport  Port=2
  eta : Inport  Port=3
  Tin : Inport  Port=4
  Add : Sum  Inputs=+-
  Add1 : Sum
  Constant : Constant
  Divide : Product  Inputs=/*
  Fcn : Fcn  Expr=u[1]^(u[2])
  K : Subsystem
  K1 : Constant  Value=1.35
  Mux : Mux  Inputs=2
  Product : Product  Inputs=4  RndMeth=Zero
  Product1 : Product  RndMeth=Zero
  Scope3 : Scope
      settings: YMin=2829.54  YMax=3127.38  SaveName=ScopeData18
  m : Fcn  Expr=(u-1)/u
  Tout : Outport
  Nout : Outport  Port=2
  wires:
  Tin/1 -> K/1(T1), Product1/2, Product/4
  Pi/1 -> Mux/1
  m/1 -> Mux/2
  Mux/1 -> Fcn/1
  Fcn/1 -> Add/1
  Add/1 -> Divide/2
  Divide/1 -> Add1/1, Product/1
  Constant/1 -> Add/2, Add1/2
  Product1/1 -> Tout/1, Scope3/1
  Product/1 -> Nout/1
  Add1/1 -> Product1/1
  K/2(Cp) -> Product/2
  Gin/1 -> Product/3
  eta/1 -> Divide/1
  K1/1 -> m/1

== system ranqilunji/HC/zhehe ==
  n : Inport
  Tin : Inport  Port=2
  Divide : Product  Inputs=*/
  Fcn : Fcn  Expr=sqrt(u/288)
  nz : Outport
  wires:
  Tin/1 -> Fcn/1
  n/1 -> Divide/1
  Fcn/1 -> Divide/2
  Divide/1 -> nz/1

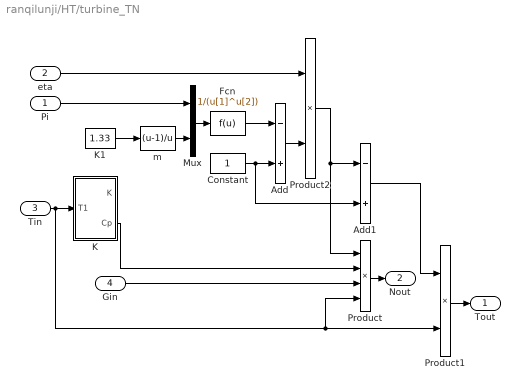
== system ranqilunji/HT/turbine_TN ==
  Pi : Inport
  eta : Inport  Port=2
  Tin : Inport  Port=3
  Gin : Inport  Port=4
  Add : Sum  Inputs=-+
  Add1 : Sum  Inputs=-+
  Constant : Constant
  Fcn : Fcn  Expr=1/(u[1]^u[2])
  K : Subsystem
  K1 : Constant  Value=1.33
  Mux : Mux  Inputs=2
  Product : Product  Inputs=4  RndMeth=Zero
  Product1 : Product  RndMeth=Zero
  Product2 : Product  RndMeth=Zero
  m : Fcn  Expr=(u-1)/u
  Tout : Outport
  Nout : Outport  Port=2
  wires:
  Tin/1 -> K/1(T1), Product1/2, Product/4
  Pi/1 -> Mux/1
  m/1 -> Mux/2
  Mux/1 -> Fcn/1
  Fcn/1 -> Add/1
  Add/1 -> Product2/2
  eta/1 -> Product2/1
  Product2/1 -> Add1/1, Product/1
  Constant/1 -> Add/2, Add1/2
  Product1/1 -> Tout/1
  Product/1 -> Nout/1
  Add1/1 -> Product1/1
  K/2(Cp) -> Product/2
  Gin/1 -> Product/3
  K1/1 -> m/1

== system ranqilunji/LC/Subsystem1 ==
  Gin : Inport
  Pin : Inport  Port=2
  Tin : Inport  Port=3
  Divide : Product  Inputs=*/
  Divide1 : Product  Inputs=*/
  Divide2 : Product  Inputs=*/
  Fcn : Fcn  Expr=sqrt(u)
  P0 : Constant  Value=100000
  Product : Product  RndMeth=Zero
  T0 : Constant  Value=288
  Gz : Outport
  wires:
  Tin/1 -> Divide/1
  T0/1 -> Divide/2
  Divide/1 -> Fcn/1
  Pin/1 -> Divide1/1
  P0/1 -> Divide1/2
  Gin/1 -> Divide2/1
  Divide1/1 -> Divide2/2
  Fcn/1 -> Product/1
  Divide2/1 -> Product/2
  Product/1 -> Gz/1

== system ranqilunji/LC/Subsystem3 ==
  Gz : Inport
  nz : Inport  Port=2
  Lookup Table (2-D) : Lookup2D  RowIndex=[4300 5000 5500 6000 6500 7000 7500 8000]  ColumnIndex=[20:0.5:100]  Table=|
      | [1.1111 1.1471 1.1832 1.2192 1.2552 1.2913 1.3273 1.3633 1.3994 1.4354 1.4714 1.5074 1.5435 1.5795 1.6155 1.6516 1.6876 1.7236 1.8750 1.8749 1.8720 1.8623 1.8457 1.8223 1.7920 1.7549 1.7109 1.6601 1.6024 1.5378 1.4664 1.3881 1.2420 1.2701 1.2983 1.3265 1.3547 1.3828 1.4110 1.4392 1.4673 1.4955 1.5237 1.5519 1.5800 1.6082 1.6364 1.6645 1.6927 1.7209 1.7491 1.7772 1.8054 1.8336 1.8617 1.8899 1.9181 1.9463 1.9744 2.0026 2.0308 2.0590 2.0871 2.1153 2.1435 2.1716 2.1998 2.2280 2.2562 2.2843 2.3125 2.3407 2.3688 2.3970 2.4252 2.4534 2.4815 2.5097 2.5379 2.5660 2.5942 2.6224 2.6506 2.6787 2.7069 2.7351 2.7633 2.7914 2.8196 2.8478 2.8759 2.9041 2.9323 2.9605 2.9886 3.0168 3.0450 3.0731 3.1013 3.1295 3.1577 3.1858 3.2140 3.2422 3.2703 3.2985 3.3267 3.3549 3.3830 3.4112 3.4394 3.4676 3.4957 3.5239 3.5521 3.5802 3.6084 3.6366 3.6648 3.6929 3.7211 3.7493 3.7774 3.8056 3.8338 3.8620 3.8901 3.9183 3.9465 3.9746 4.0028 4.0310 4.0592 4.0873 4.1155 4.1437 4.1719 4.2000 4.2282 4.2564 4.2845 4.3127 4.3409 4.3691 4.3972 4.4254 4.4536 4.4817 4.5099 4.5381 4.5663 4.5944 4.6226 4.6508 4.6789 4.7071 4.7353 4.7635 4.7916 4.8198 4.8480;
      | 1.1111 1.1471 1.1832 1.2192 1.2552 1.2913 1.3273 1.3633 1.3994 1.4354 1.4714 1.5074 1.5435 1.5795 1.6155 1.6516 1.6876 1.7236 1.7597 1.7957 1.8317 1.8678 1.9038 1.9398 1.9758 2.0119 2.0479 2.0839 2.1200 2.1560 2.1920 2.2281 2.2641 2.3001 2.3361 2.3722 2.4082 2.4442 2.4803 2.5163 2.5523 2.5884 2.5200 2.4780 2.3700 2.2800 2.1500 1.8820 1.6080 1.7209 1.7491 1.7772 1.8054 1.8336 1.8617 1.8899 1.9181 1.9463 1.9744 2.0026 2.0308 2.0590 2.0871 2.1153 2.1435 2.1716 2.1998 2.2280 2.2562 2.2843 2.3125 2.3407 2.3688 2.3970 2.4252 2.4534 2.4815 2.5097 2.5379 2.5660 2.5942 2.6224 2.6506 2.6787 2.7069 2.7351 2.7633 2.7914 2.8196 2.8478 2.8759 2.9041 2.9323 2.9605 2.9886 3.0168 3.0450 3.0731 3.1013 3.1295 3.1577 3.1858 3.2140 3.2422 3.2703 3.2985 3.3267 3.3549 3.3830 3.4112 3.4394 3.4676 3.4957 3.5239 3.5521 3.5802 3.6084 3.6366 3.6648 3.6929 3.7211 3.7493 3.7774 3.8056 3.8338 3.8620 3.8901 3.9183 3.9465 3.9746 4.0028 4.0310 4.0592 4.0873 4.1155 4.1437 4.1719 4.2000 4.2282 4.2564 4.2845 4.3127 4.3409 4.3691 4.3972 4.4254 4.4536 4.4817 4.5099 4.5381 4.5663 4.5944 4.6226 4.6508 4.6789 4.7071 4.7353 4.7635 4.7916 4.8198 4.8480;
      | 1.1111 1.1471 1.1832 1.2192 1.2552 1.2913 1.3273 1.3633 1.3994 1.4354 1.4714 1.5074 1.5435 1.5795 1.6155 1.6516 1.6876 1.7236 1.7597 1.7957 1.8317 1.8678 1.9038 1.9398 1.9758 2.0119 2.0479 2.0839 2.1200 2.1560 2.1920 2.2281 2.2641 2.3001 2.3361 2.3722 2.4082 2.4442 2.4803 2.5163 2.5523 2.5884 2.6244 2.6604 2.6965 2.7325 2.7685 2.8045 2.8406 2.8766 2.9126 2.9487 2.9847 3.0207 2.8905 2.8292 2.7444 2.6661 2.5443 2.4489 2.3700 2.1776 2.0217 2.1153 2.1435 2.1716 2.1998 2.2280 2.2562 2.2843 2.3125 2.3407 2.3688 2.3970 2.4252 2.4534 2.4815 2.5097 2.5379 2.5660 2.5942 2.6224 2.6506 2.6787 2.7069 2.7351 2.7633 2.7914 2.8196 2.8478 2.8759 2.9041 2.9323 2.9605 2.9886 3.0168 3.0450 3.0731 3.1013 3.1295 3.1577 3.1858 3.2140 3.2422 3.2703 3.2985 3.3267 3.3549 3.3830 3.4112 3.4394 3.4676 3.4957 3.5239 3.5521 3.5802 3.6084 3.6366 3.6648 3.6929 3.7211 3.7493 3.7774 3.8056 3.8338 3.8620 3.8901 3.9183 3.9465 3.9746 4.0028 4.0310 4.0592 4.0873 4.1155 4.1437 4.1719 4.2000 4.2282 4.2564 4.2845 4.3127 4.3409 4.3691 4.3972 4.4254 4.4536 4.4817 4.5099 4.5381 4.5663 4.5944 4.6226 4.6508 4.6789 4.7071 4.7353 4.7635 4.7916 4.8198 4.8480;
      | 1.1111 1.1471 1.1832 1.2192 1.2552 1.2913 1.3273 1.3633 1.3994 1.4354 1.4714 1.5074 1.5435 1.5795 1.6155 1.6516 1.6876 1.7236 1.7597 1.7957 1.8317 1.8678 1.9038 1.9398 1.9758 2.0119 2.0479 2.0839 2.1200 2.1560 2.1920 2.2281 2.2641 2.3001 2.3361 2.3722 2.4082 2.4442 2.4803 2.5163 2.5523 2.5884 2.6244 2.6604 2.6965 2.7325 2.7685 2.8045 2.8406 2.8766 2.9126 2.9487 2.9847 3.0207 3.0568 3.0928 3.1288 3.1648 3.2009 3.2369 3.2729 3.3090 3.3450 3.3810 3.3655 3.3396 3.3040 3.2587 3.2037 3.1389 3.0645 2.9803 2.8865 2.7829 2.6696 2.5466 2.4815 2.5097 2.5379 2.5660 2.5942 2.6224 2.6506 2.6787 2.7069 2.7351 2.7633 2.7914 2.8196 2.8478 2.8759 2.9041 2.9323 2.9605 2.9886 3.0168 3.0450 3.0731 3.1013 3.1295 3.1577 3.1858 3.2140 3.2422 3.2703 3.2985 3.3267 3.3549 3.3830 3.4112 3.4394 3.4676 3.4957 3.5239 3.5521 3.5802 3.6084 3.6366 3.6648 3.6929 3.7211 3.7493 3.7774 3.8056 3.8338 3.8620 3.8901 3.9183 3.9465 3.9746 4.0028 4.0310 4.0592 4.0873 4.1155 4.1437 4.1719 4.2000 4.2282 4.2564 4.2845 4.3127 4.3409 4.3691 4.3972 4.4254 4.4536 4.4817 4.5099 4.5381 4.5663 4.5944 4.6226 4.6508 4.6789 4.7071 4.7353 4.7635 4.7916 4.8198 4.8480;
      | 1.1111 1.1471 1.1832 1.2192 1.2552 1.2913 1.3273 1.3633 1.3994 1.4354 1.4714 1.5074 1.5435 1.5795 1.6155 1.6516 1.6876 1.7236 1.7597 1.7957 1.8317 1.8678 1.9038 1.9398 1.9758 2.0119 2.0479 2.0839 2.1200 2.1560 2.1920 2.2281 2.2641 2.3001 2.3361 2.3722 2.4082 2.4442 2.4803 2.5163 2.5523 2.5884 2.6244 2.6604 2.6965 2.7325 2.7685 2.8045 2.8406 2.8766 2.9126 2.9487 2.9847 3.0207 3.0568 3.0928 3.1288 3.1648 3.2009 3.2369 3.2729 3.3090 3.3450 3.3810 3.4171 3.4531 3.4891 3.5252 3.5612 3.5972 3.6332 3.6693 3.7053 3.7413 3.7774 3.8134 3.8494 3.8855 3.9215 3.9575 3.9936 4.0296 4.0656 4.1016 4.1377 4.1737 4.2097 4.2458 4.2818 4.3178 4.3646 4.3478 4.3218 4.2866 4.2421 4.1884 4.1254 4.0533 3.9718 3.8812 3.7813 3.6722 3.5538 3.4262 3.2894 3.2985 3.3267 3.3549 3.3830 3.4112 3.4394 3.4676 3.4957 3.5239 3.5521 3.5802 3.6084 3.6366 3.6648 3.6929 3.7211 3.7493 3.7774 3.8056 3.8338 3.8620 3.8901 3.9183 3.9465 3.9746 4.0028 4.0310 4.0592 4.0873 4.1155 4.1437 4.1719 4.2000 4.2282 4.2564 4.2845 4.3127 4.3409 4.3691 4.3972 4.4254 4.4536 4.4817 4.5099 4.5381 4.5663 4.5944 4.6226 4.6508 4.6789 4.7071 4.7353 4.7635 4.7916 4.8198 4.8480;
      | 1.1111 1.1471 1.1832 1.2192 1.2552 1.2913 1.3273 1.3633 1.3994 1.4354 1.4714 1.5074 1.5435 1.5795 1.6155 1.6516 1.6876 1.7236 1.7597 1.7957 1.8317 1.8678 1.9038 1.9398 1.9758 2.0119 2.0479 2.0839 2.1200 2.1560 2.1920 2.2281 2.2641 2.3001 2.3361 2.3722 2.4082 2.4442 2.4803 2.5163 2.5523 2.5884 2.6244 2.6604 2.6965 2.7325 2.7685 2.8045 2.8406 2.8766 2.9126 2.9487 2.9847 3.0207 3.0568 3.0928 3.1288 3.1648 3.2009 3.2369 3.2729 3.3090 3.3450 3.3810 3.4171 3.4531 3.4891 3.5252 3.5612 3.5972 3.6332 3.6693 3.7053 3.7413 3.7774 3.8134 3.8494 3.8855 3.9215 3.9575 3.9936 4.0296 4.0656 4.1016 4.1377 4.1737 4.2097 4.2458 4.2818 4.3178 4.3539 4.3899 4.4259 4.4619 4.4980 4.5340 4.5700 4.6061 4.6421 4.6781 4.7142 4.7502 4.7862 4.8223 4.8583 4.8943 4.9303 4.9664 5.0024 5.0384 5.0745 5.1105 5.1465 5.3241 5.3091 5.2474 5.1391 4.9841 4.7824 4.5341 4.2392 3.8976 3.7774 3.8056 3.8338 3.8620 3.8901 3.9183 3.9465 3.9746 4.0028 4.0310 4.0592 4.0873 4.1155 4.1437 4.1719 4.2000 4.2282 4.2564 4.2845 4.3127 4.3409 4.3691 4.3972 4.4254 4.4536 4.4817 4.5099 4.5381 4.5663 4.5944 4.6226 4.6508 4.6789 4.7071 4.7353 4.7635 4.7916 4.8198 4.8480;
      | 1.1111 1.1471 1.1832 1.2192 1.2552 1.2913 1.3273 1.3633 1.3994 1.4354 1.4714 1.5074 1.5435 1.5795 1.6155 1.6516 1.6876 1.7236 1.7597 1.7957 1.8317 1.8678 1.9038 1.9398 1.9758 2.0119 2.0479 2.0839 2.1200 2.1560 2.1920 2.2281 2.2641 2.3001 2.3361 2.3722 2.4082 2.4442 2.4803 2.5163 2.5523 2.5884 2.6244 2.6604 2.6965 2.7325 2.7685 2.8045 2.8406 2.8766 2.9126 2.9487 2.9847 3.0207 3.0568 3.0928 3.1288 3.1648 3.2009 3.2369 3.2729 3.3090 3.3450 3.3810 3.4171 3.4531 3.4891 3.5252 3.5612 3.5972 3.6332 3.6693 3.7053 3.7413 3.7774 3.8134 3.8494 3.8855 3.9215 3.9575 3.9936 4.0296 4.0656 4.1016 4.1377 4.1737 4.2097 4.2458 4.2818 4.3178 4.3539 4.3899 4.4259 4.4619 4.4980 4.5340 4.5700 4.6061 4.6421 4.6781 4.7142 4.7502 4.7862 4.8223 4.8583 4.8943 4.9303 4.9664 5.0024 5.0384 5.0745 5.1105 5.1465 5.1826 5.2186 5.2546 5.2906 5.3267 5.3627 5.3987 5.4348 5.4708 5.5068 5.5429 5.5789 5.6149 5.6510 5.6870 5.7230 5.7590 5.7951 5.8311 5.8671 5.9032 5.9392 5.9752 6.0113 6.0473 5.2600 4.2400 4.2845 4.3127 4.3409 4.3691 4.3972 4.4254 4.4536 4.4817 4.5099 4.5381 4.5663 4.5944 4.6226 4.6508 4.6789 4.7071 4.7353 4.7635 4.7916 4.8198 4.8480;
      | 1.1111 1.1471 1.1832 1.2192 1.2552 1.2913 1.3273 1.3633 1.3994 1.4354 1.4714 1.5074 1.5435 1.5795 1.6155 1.6516 1.6876 1.7236 1.7597 1.7957 1.8317 1.8678 1.9038 1.9398 1.9758 2.0119 2.0479 2.0839 2.1200 2.1560 2.1920 2.2281 2.2641 2.3001 2.3361 2.3722 2.4082 2.4442 2.4803 2.5163 2.5523 2.5884 2.6244 2.6604 2.6965 2.7325 2.7685 2.8045 2.8406 2.8766 2.9126 2.9487 2.9847 3.0207 3.0568 3.0928 3.1288 3.1648 3.2009 3.2369 3.2729 3.3090 3.3450 3.3810 3.4171 3.4531 3.4891 3.5252 3.5612 3.5972 3.6332 3.6693 3.7053 3.7413 3.7774 3.8134 3.8494 3.8855 3.9215 3.9575 3.9936 4.0296 4.0656 4.1016 4.1377 4.1737 4.2097 4.2458 4.2818 4.3178 4.3539 4.3899 4.4259 4.4619 4.4980 4.5340 4.5700 4.6061 4.6421 4.6781 4.7142 4.7502 4.7862 4.8223 4.8583 4.8943 4.9303 4.9664 5.0024 5.0384 5.0745 5.1105 5.1465 5.1826 5.2186 5.2546 5.2906 5.3267 5.3627 5.3987 5.4348 5.4708 5.5068 5.5429 5.5789 5.6149 5.6510 5.6870 5.7230 5.7590 5.7951 5.8311 5.8671 5.9032 5.9392 5.9752 6.0113 6.0473 6.0833 6.1193 6.1554 6.1914 6.2274 6.2635 6.2995 6.3355 6.3716 6.4076 6.4436 6.4797 6.5157 6.5517 6.5877 6.6238 6.6598 4.7071 4.7353 4.7635 4.7916 4.8198 4.8480;]
  Lookup Table (2-D)1 : Lookup2D  RowIndex=[4300 5000 5500 6000 6500 7000 7500 8000]  ColumnIndex=[20:0.5:100]  Table=|
      | [0.8303 0.8307 0.8310 0.8314 0.8317 0.8321 0.8324 0.8327 0.8331 0.8335 0.8338 0.8341 0.8345 0.8348 0.8351 0.8355 0.8358 0.8361 0.8371 0.8390 0.8403 0.8412 0.8415 0.8412 0.8405 0.8392 0.8373 0.8350 0.8321 0.8287 0.8247 0.8203 0.8200 0.8200 0.8200 0.8200 0.8200 0.8200 0.8200 0.8200 0.8200 0.8200 0.8200 0.8200 0.8200 0.8200 0.8200 0.8200 0.8200 0.8200 0.8200 0.8200 0.8200 0.8200 0.8200 0.8200 0.8200 0.8200 0.8200 0.8200 0.8200 0.8200 0.8200 0.8200 0.8200 0.8200 0.8200 0.8200 0.8200 0.8200 0.8200 0.8200 0.8200 0.8200 0.8200 0.8200 0.8200 0.8200 0.8200 0.8200 0.8200 0.8200 0.8200 0.8200 0.8200 0.8200 0.8200 0.8200 0.8200 0.8200 0.8200 0.8200 0.8200 0.8200 0.8200 0.8200 0.8200 0.8200 0.8200 0.8200 0.8200 0.8200 0.8200 0.8200 0.8200 0.8500 0.8500 0.8500 0.8500 0.8500 0.8500 0.8500 0.8500 0.8500 0.8500 0.8500 0.8500 0.8500 0.8500 0.8500 0.8500 0.8500 0.8500 0.8500 0.8500 0.8500 0.8500 0.8500 0.8500 0.8500 0.8500 0.8500 0.8500 0.8500 0.8500 0.8500 0.8500 0.8500 0.8500 0.8500 0.8500 0.8500 0.8500 0.8500 0.8500 0.8500 0.8500 0.8500 0.8500 0.8500 0.8500 0.8500 0.8500 0.8500 0.8500 0.8500 0.8500 0.8500 0.8500 0.8500 0.8500;
      | 0.8303 0.8307 0.8310 0.8314 0.8317 0.8321 0.8324 0.8327 0.8331 0.8335 0.8338 0.8341 0.8345 0.8348 0.8351 0.8355 0.8358 0.8361 0.8371 0.8375 0.8379 0.8383 0.8387 0.8391 0.8395 0.8400 0.8402 0.8405 0.8407 0.8410 0.8412 0.8415 0.8417 0.8420 0.8422 0.8425 0.8427 0.8430 0.8432 0.8435 0.8437 0.8440 0.8441 0.8727 0.8851 0.8814 0.8616 0.8257 0.8200 0.8200 0.8200 0.8200 0.8200 0.8200 0.8200 0.8200 0.8200 0.8200 0.8200 0.8200 0.8200 0.8200 0.8200 0.8200 0.8200 0.8200 0.8200 0.8200 0.8200 0.8200 0.8200 0.8200 0.8200 0.8200 0.8200 0.8200 0.8200 0.8200 0.8200 0.8200 0.8200 0.8200 0.8200 0.8200 0.8200 0.8200 0.8200 0.8200 0.8200 0.8200 0.8200 0.8200 0.8200 0.8200 0.8200 0.8200 0.8200 0.8200 0.8200 0.8200 0.8200 0.8200 0.8200 0.8200 0.8200 0.8500 0.8500 0.8500 0.8500 0.8500 0.8500 0.8500 0.8500 0.8500 0.8500 0.8500 0.8500 0.8500 0.8500 0.8500 0.8500 0.8500 0.8500 0.8500 0.8500 0.8500 0.8500 0.8500 0.8500 0.8500 0.8500 0.8500 0.8500 0.8500 0.8500 0.8500 0.8500 0.8500 0.8500 0.8500 0.8500 0.8500 0.8500 0.8500 0.8500 0.8500 0.8500 0.8500 0.8500 0.8500 0.8500 0.8500 0.8500 0.8500 0.8500 0.8500 0.8500 0.8500 0.8500 0.8500 0.8500;
      | 0.8303 0.8307 0.8310 0.8314 0.8317 0.8321 0.8324 0.8327 0.8331 0.8335 0.8338 0.8341 0.8345 0.8348 0.8351 0.8355 0.8358 0.8361 0.8371 0.8375 0.8379 0.8383 0.8387 0.8391 0.8395 0.8400 0.8402 0.8405 0.8407 0.8410 0.8412 0.8415 0.8417 0.8420 0.8422 0.8425 0.8427 0.8430 0.8432 0.8435 0.8437 0.8440 0.8441 0.8440 0.8440 0.8440 0.8440 0.8440 0.8400 0.8400 0.8400 0.8400 0.8400 0.8400 0.8400 0.8400 0.8420 0.8439 0.8592 0.8652 0.8619 0.8495 0.8278 0.8200 0.8200 0.8200 0.8200 0.8200 0.8200 0.8200 0.8200 0.8200 0.8200 0.8200 0.8200 0.8200 0.8200 0.8200 0.8200 0.8200 0.8200 0.8200 0.8200 0.8200 0.8200 0.8200 0.8200 0.8200 0.8200 0.8200 0.8200 0.8200 0.8200 0.8200 0.8200 0.8200 0.8200 0.8200 0.8200 0.8200 0.8200 0.8200 0.8200 0.8200 0.8200 0.8500 0.8500 0.8500 0.8500 0.8500 0.8500 0.8500 0.8500 0.8500 0.8500 0.8500 0.8500 0.8500 0.8500 0.8500 0.8500 0.8500 0.8500 0.8500 0.8500 0.8500 0.8500 0.8500 0.8500 0.8500 0.8500 0.8500 0.8500 0.8500 0.8500 0.8500 0.8500 0.8500 0.8500 0.8500 0.8500 0.8500 0.8500 0.8500 0.8500 0.8500 0.8500 0.8500 0.8500 0.8500 0.8500 0.8500 0.8500 0.8500 0.8500 0.8500 0.8500 0.8500 0.8500 0.8500 0.8500;
      | 0.8303 0.8307 0.8310 0.8314 0.8317 0.8321 0.8324 0.8327 0.8331 0.8335 0.8338 0.8341 0.8345 0.8348 0.8351 0.8355 0.8358 0.8361 0.8371 0.8375 0.8379 0.8383 0.8387 0.8391 0.8395 0.8400 0.8402 0.8405 0.8407 0.8410 0.8412 0.8415 0.8417 0.8420 0.8422 0.8425 0.8427 0.8430 0.8432 0.8435 0.8437 0.8440 0.8441 0.8440 0.8440 0.8440 0.8440 0.8440 0.8400 0.8400 0.8400 0.8400 0.8400 0.8400 0.8400 0.8390 0.8380 0.8370 0.8360 0.8350 0.8340 0.8330 0.8320 0.8310 0.8300 0.8300 0.8300 0.8371 0.8489 0.8568 0.8608 0.8609 0.8570 0.8492 0.8375 0.8219 0.8200 0.8200 0.8200 0.8200 0.8200 0.8200 0.8200 0.8200 0.8200 0.8200 0.8200 0.8200 0.8200 0.8200 0.8200 0.8200 0.8200 0.8200 0.8200 0.8200 0.8200 0.8200 0.8200 0.8200 0.8200 0.8200 0.8200 0.8200 0.8200 0.8500 0.8500 0.8500 0.8500 0.8500 0.8500 0.8500 0.8500 0.8500 0.8500 0.8500 0.8500 0.8500 0.8500 0.8500 0.8500 0.8500 0.8500 0.8500 0.8500 0.8500 0.8500 0.8500 0.8500 0.8500 0.8500 0.8500 0.8500 0.8500 0.8500 0.8500 0.8500 0.8500 0.8500 0.8500 0.8500 0.8500 0.8500 0.8500 0.8500 0.8500 0.8500 0.8500 0.8500 0.8500 0.8500 0.8500 0.8500 0.8500 0.8500 0.8500 0.8500 0.8500 0.8500 0.8500 0.8500;
      | 0.8303 0.8307 0.8310 0.8314 0.8317 0.8321 0.8324 0.8327 0.8331 0.8335 0.8338 0.8341 0.8345 0.8348 0.8351 0.8355 0.8358 0.8361 0.8371 0.8375 0.8379 0.8383 0.8387 0.8391 0.8395 0.8400 0.8402 0.8405 0.8407 0.8410 0.8412 0.8415 0.8417 0.8420 0.8422 0.8425 0.8427 0.8430 0.8432 0.8435 0.8437 0.8440 0.8441 0.8440 0.8440 0.8440 0.8440 0.8440 0.8400 0.8400 0.8400 0.8400 0.8400 0.8400 0.8400 0.8390 0.8380 0.8370 0.8360 0.8350 0.8340 0.8330 0.8320 0.8310 0.8300 0.8306 0.8312 0.8318 0.8324 0.8330 0.8336 0.8342 0.8348 0.8354 0.8360 0.8366 0.8372 0.8378 0.8384 0.8390 0.8396 0.8402 0.8408 0.8414 0.8420 0.8426 0.8432 0.8435 0.8438 0.8442 0.8438 0.8515 0.8581 0.8636 0.8680 0.8712 0.8733 0.8743 0.8742 0.8730 0.8706 0.8671 0.8625 0.8568 0.8500 0.8500 0.8500 0.8500 0.8500 0.8500 0.8500 0.8500 0.8500 0.8500 0.8500 0.8500 0.8500 0.8500 0.8500 0.8500 0.8500 0.8500 0.8500 0.8500 0.8500 0.8500 0.8500 0.8500 0.8500 0.8500 0.8500 0.8500 0.8500 0.8500 0.8500 0.8500 0.8500 0.8500 0.8500 0.8500 0.8500 0.8500 0.8500 0.8500 0.8500 0.8500 0.8500 0.8500 0.8500 0.8500 0.8500 0.8500 0.8500 0.8500 0.8500 0.8500 0.8500 0.8500 0.8500 0.8500 0.8500;
      | 0.8303 0.8307 0.8310 0.8314 0.8317 0.8321 0.8324 0.8327 0.8331 0.8335 0.8338 0.8341 0.8345 0.8348 0.8351 0.8355 0.8358 0.8361 0.8371 0.8375 0.8379 0.8383 0.8387 0.8391 0.8395 0.8400 0.8402 0.8405 0.8407 0.8410 0.8412 0.8415 0.8417 0.8420 0.8422 0.8425 0.8427 0.8430 0.8432 0.8435 0.8437 0.8440 0.8441 0.8440 0.8440 0.8440 0.8440 0.8440 0.8400 0.8400 0.8400 0.8400 0.8400 0.8400 0.8400 0.8390 0.8380 0.8370 0.8360 0.8350 0.8340 0.8330 0.8320 0.8310 0.8300 0.8306 0.8312 0.8318 0.8324 0.8330 0.8336 0.8342 0.8348 0.8354 0.8360 0.8366 0.8372 0.8378 0.8384 0.8390 0.8396 0.8402 0.8408 0.8414 0.8420 0.8426 0.8432 0.8435 0.8438 0.8442 0.8448 0.8452 0.8457 0.8462 0.8467 0.8472 0.8476 0.8451 0.8486 0.8491 0.8496 0.8500 0.8505 0.8510 0.8515 0.8520 0.8524 0.8529 0.8534 0.8539 0.8544 0.8548 0.8549 0.8550 0.8600 0.8650 0.8746 0.8872 0.8921 0.8890 0.8782 0.8595 0.8500 0.8500 0.8500 0.8500 0.8500 0.8500 0.8500 0.8500 0.8500 0.8500 0.8500 0.8500 0.8500 0.8500 0.8500 0.8500 0.8500 0.8500 0.8500 0.8500 0.8500 0.8500 0.8500 0.8500 0.8500 0.8500 0.8500 0.8500 0.8500 0.8500 0.8500 0.8500 0.8500 0.8500 0.8500 0.8500 0.8500 0.8500 0.8500;
      | 0.8303 0.8307 0.8310 0.8314 0.8317 0.8321 0.8324 0.8327 0.8331 0.8335 0.8338 0.8341 0.8345 0.8348 0.8351 0.8355 0.8358 0.8361 0.8371 0.8375 0.8379 0.8383 0.8387 0.8391 0.8395 0.8400 0.8402 0.8405 0.8407 0.8410 0.8412 0.8415 0.8417 0.8420 0.8422 0.8425 0.8427 0.8430 0.8432 0.8435 0.8437 0.8440 0.8441 0.8440 0.8440 0.8440 0.8440 0.8440 0.8400 0.8400 0.8400 0.8400 0.8400 0.8400 0.8400 0.8390 0.8380 0.8370 0.8360 0.8350 0.8340 0.8330 0.8320 0.8310 0.8300 0.8306 0.8312 0.8318 0.8324 0.8330 0.8336 0.8342 0.8348 0.8354 0.8360 0.8366 0.8372 0.8378 0.8384 0.8390 0.8396 0.8402 0.8408 0.8414 0.8420 0.8426 0.8432 0.8435 0.8438 0.8442 0.8448 0.8452 0.8457 0.8462 0.8467 0.8472 0.8476 0.8451 0.8486 0.8491 0.8496 0.8500 0.8505 0.8510 0.8515 0.8520 0.8524 0.8529 0.8534 0.8539 0.8544 0.8548 0.8549 0.8550 0.8550 0.8550 0.8550 0.8550 0.8550 0.8550 0.8550 0.8550 0.8550 0.8550 0.8550 0.8550 0.8550 0.8550 0.8550 0.8550 0.8550 0.8550 0.8550 0.8550 0.8550 0.8550 0.8550 0.8550 0.8788 0.8500 0.8500 0.8500 0.8500 0.8500 0.8500 0.8500 0.8500 0.8500 0.8500 0.8500 0.8500 0.8500 0.8500 0.8500 0.8500 0.8500 0.8500 0.8500 0.8500 0.8500 0.8500;
      | 0.8303 0.8307 0.8310 0.8314 0.8317 0.8321 0.8324 0.8327 0.8331 0.8335 0.8338 0.8341 0.8345 0.8348 0.8351 0.8355 0.8358 0.8361 0.8371 0.8375 0.8379 0.8383 0.8387 0.8391 0.8395 0.8400 0.8402 0.8405 0.8407 0.8410 0.8412 0.8415 0.8417 0.8420 0.8422 0.8425 0.8427 0.8430 0.8432 0.8435 0.8437 0.8440 0.8441 0.8440 0.8440 0.8440 0.8440 0.8440 0.8400 0.8400 0.8400 0.8400 0.8400 0.8400 0.8400 0.8390 0.8380 0.8370 0.8360 0.8350 0.8340 0.8330 0.8320 0.8310 0.8300 0.8306 0.8312 0.8318 0.8324 0.8330 0.8336 0.8342 0.8348 0.8354 0.8360 0.8366 0.8372 0.8378 0.8384 0.8390 0.8396 0.8402 0.8408 0.8414 0.8420 0.8426 0.8432 0.8435 0.8438 0.8442 0.8448 0.8452 0.8457 0.8462 0.8467 0.8472 0.8476 0.8451 0.8486 0.8491 0.8496 0.8500 0.8505 0.8510 0.8515 0.8520 0.8524 0.8529 0.8534 0.8539 0.8544 0.8548 0.8549 0.8550 0.8550 0.8550 0.8550 0.8550 0.8550 0.8550 0.8550 0.8550 0.8550 0.8550 0.8550 0.8550 0.8550 0.8550 0.8550 0.8550 0.8550 0.8550 0.8550 0.8550 0.8550 0.8550 0.8550 0.8550 0.8550 0.8550 0.8550 0.8550 0.8550 0.8550 0.8550 0.8550 0.8550 0.8550 0.8550 0.8550 0.8550 0.8550 0.8550 0.8550 0.8550 0.8550 0.8500 0.8500 0.8500 0.8500 0.8550;]
  pi : Outport
  eta : Outport  Port=2
  wires:
  nz/1 -> Lookup Table (2-D)/1, Lookup Table (2-D)1/1
  Gz/1 -> Lookup Table (2-D)1/2, Lookup Table (2-D)/2
  Lookup Table (2-D)/1 -> pi/1
  Lookup Table (2-D)1/1 -> eta/1

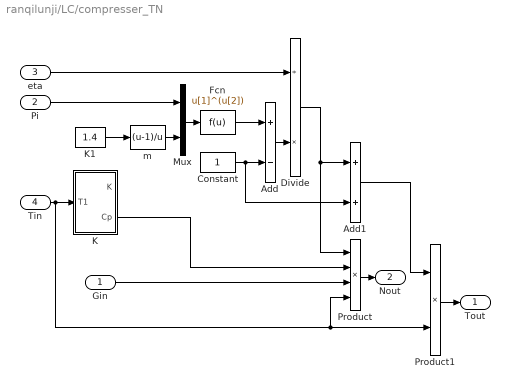
== system ranqilunji/LC/compresser_TN ==
  Gin : Inport
  Pi : Inport  Port=2
  eta : Inport  Port=3
  Tin : Inport  Port=4
  Add : Sum  Inputs=+-
  Add1 : Sum
  Constant : Constant
  Divide : Product  Inputs=/*
  Fcn : Fcn  Expr=u[1]^(u[2])
  K : Subsystem
  K1 : Constant  Value=1.4
  Mux : Mux  Inputs=2
  Product : Product  Inputs=4  RndMeth=Zero
  Product1 : Product  RndMeth=Zero
  m : Fcn  Expr=(u-1)/u
  Tout : Outport
  Nout : Outport  Port=2
  wires:
  Tin/1 -> K/1(T1), Product1/2, Product/4
  Pi/1 -> Mux/1
  m/1 -> Mux/2
  Mux/1 -> Fcn/1
  Fcn/1 -> Add/1
  Add/1 -> Divide/2
  eta/1 -> Divide/1
  Divide/1 -> Add1/1, Product/1
  Constant/1 -> Add/2, Add1/2
  Product1/1 -> Tout/1
  Product/1 -> Nout/1
  Add1/1 -> Product1/1
  K/2(Cp) -> Product/2
  Gin/1 -> Product/3
  K1/1 -> m/1

== system ranqilunji/LC/zhehe ==
  n : Inport
  Tin : Inport  Port=2
  Divide : Product  Inputs=*/
  Fcn : Fcn  Expr=sqrt(u/288)
  nz : Outport
  wires:
  Tin/1 -> Fcn/1
  n/1 -> Divide/1
  Fcn/1 -> Divide/2
  Divide/1 -> nz/1

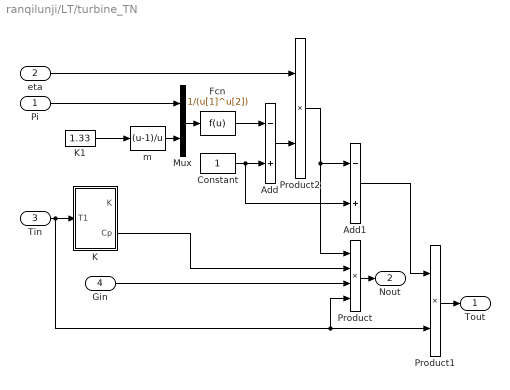
== system ranqilunji/LT/turbine_TN ==
  Pi : Inport
  eta : Inport  Port=2
  Tin : Inport  Port=3
  Gin : Inport  Port=4
  Add : Sum  Inputs=-+
  Add1 : Sum  Inputs=-+
  Constant : Constant
  Fcn : Fcn  Expr=1/(u[1]^u[2])
  K : Subsystem
  K1 : Constant  Value=1.33
  Mux : Mux  Inputs=2
  Product : Product  Inputs=4  RndMeth=Zero
  Product1 : Product  RndMeth=Zero
  Product2 : Product  RndMeth=Zero
  m : Fcn  Expr=(u-1)/u
  Tout : Outport
  Nout : Outport  Port=2
  wires:
  Tin/1 -> K/1(T1), Product1/2, Product/4
  Pi/1 -> Mux/1
  m/1 -> Mux/2
  Mux/1 -> Fcn/1
  Fcn/1 -> Add/1
  Add/1 -> Product2/2
  eta/1 -> Product2/1
  Product2/1 -> Add1/1, Product/1
  Constant/1 -> Add/2, Add1/2
  Product1/1 -> Tout/1
  Product/1 -> Nout/1
  Add1/1 -> Product1/1
  K/2(Cp) -> Product/2
  Gin/1 -> Product/3
  K1/1 -> m/1

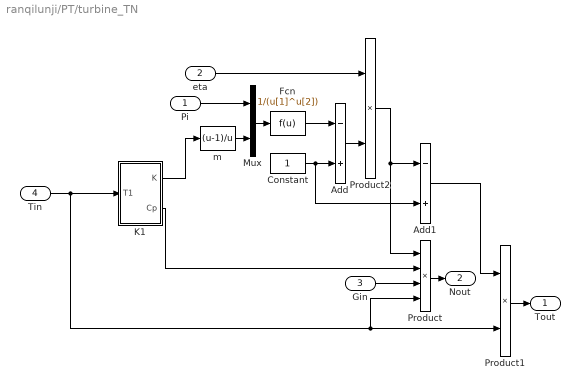
== system ranqilunji/PT/turbine_TN ==
  Pi : Inport
  eta : Inport  Port=2
  Gin : Inport  Port=3
  Tin : Inport  Port=4
  Add : Sum  Inputs=-+
  Add1 : Sum  Inputs=-+
  Constant : Constant
  Fcn : Fcn  Expr=1/(u[1]^u[2])
  K1 : Subsystem
  Mux : Mux  Inputs=2
  Product : Product  Inputs=4  RndMeth=Zero
  Product1 : Product  RndMeth=Zero
  Product2 : Product  RndMeth=Zero
  m : Fcn  Expr=(u-1)/u
  Tout : Outport
  Nout : Outport  Port=2
  wires:
  Pi/1 -> Mux/1
  m/1 -> Mux/2
  Mux/1 -> Fcn/1
  Fcn/1 -> Add/1
  Add/1 -> Product2/2
  eta/1 -> Product2/1
  Product2/1 -> Add1/1, Product/1
  Constant/1 -> Add/2, Add1/2
  Product1/1 -> Tout/1
  Product/1 -> Nout/1
  Add1/1 -> Product1/1
  Gin/1 -> Product/3
  Tin/1 -> K1/1(T1), Product1/2, Product/4
  K1/2(Cp) -> Product/2
  K1/1(K) -> m/1

== system ranqilunji/HC/compresser_TN/K ==
  note: Cv
  note: Cp
  T1 : Inport
  Add : Sum
  Add1 : Sum
  Add2 : Sum  Inputs=+-
  Constant : Constant  Value=0.9956
  Constant1 : Constant  Value=0.7088
  Divide1 : Product  Inputs=*/
  Gain2 : Gain  Gain=0.000093
  Gain3 : Gain  Gain=0.000093
  Scope3 : Scope
      settings: YMin=2829.54  YMax=3127.38  SaveName=ScopeData23
  Tk : Constant  Value=273.15
  K : Outport
  Cp : Outport  Port=2
  wires:
  Divide1/1 -> K/1, Scope3/1
  Add1/1 -> Divide1/2
  Constant1/1 -> Add1/2
  Gain3/1 -> Add1/1
  Add/1 -> Divide1/1, Cp/1
  Constant/1 -> Add/2
  Gain2/1 -> Add/1
  T1/1 -> Add2/1
  Tk/1 -> Add2/2
  Add2/1 -> Gain2/1, Gain3/1

== system ranqilunji/HT/turbine_TN/K ==
  note: Cv
  note: Cp
  T1 : Inport
  Add : Sum
  Add1 : Sum
  Add2 : Sum  Inputs=+-
  Constant : Constant  Value=0.9956
  Constant1 : Constant  Value=0.7088
  Divide1 : Product  Inputs=*/
  Gain2 : Gain  Gain=0.000093
  Gain3 : Gain  Gain=0.000093
  Tk : Constant  Value=273.15
  K : Outport
  Cp : Outport  Port=2
  wires:
  Divide1/1 -> K/1
  Add1/1 -> Divide1/2
  Constant1/1 -> Add1/2
  Gain3/1 -> Add1/1
  Add/1 -> Divide1/1, Cp/1
  Constant/1 -> Add/2
  Gain2/1 -> Add/1
  T1/1 -> Add2/1
  Tk/1 -> Add2/2
  Add2/1 -> Gain2/1, Gain3/1

== system ranqilunji/LC/compresser_TN/K ==
  note: Cv
  note: Cp
  T1 : Inport
  Add : Sum
  Add1 : Sum
  Add2 : Sum  Inputs=+-
  Constant : Constant  Value=0.9956
  Constant1 : Constant  Value=0.7088
  Divide1 : Product  Inputs=*/
  Gain2 : Gain  Gain=0.000093
  Gain3 : Gain  Gain=0.000093
  Tk : Constant  Value=273.15
  K : Outport
  Cp : Outport  Port=2
  wires:
  Divide1/1 -> K/1
  Add1/1 -> Divide1/2
  Constant1/1 -> Add1/2
  Gain3/1 -> Add1/1
  Add/1 -> Divide1/1, Cp/1
  Constant/1 -> Add/2
  Gain2/1 -> Add/1
  T1/1 -> Add2/1
  Tk/1 -> Add2/2
  Add2/1 -> Gain2/1, Gain3/1

== system ranqilunji/LT/turbine_TN/K ==
  note: Cv
  note: Cp
  T1 : Inport
  Add : Sum
  Add1 : Sum
  Add2 : Sum  Inputs=+-
  Constant : Constant  Value=0.9956
  Constant1 : Constant  Value=0.7088
  Divide1 : Product  Inputs=*/
  Gain2 : Gain  Gain=0.000093
  Gain3 : Gain  Gain=0.000093
  Tk : Constant  Value=273.15
  K : Outport
  Cp : Outport  Port=2
  wires:
  Divide1/1 -> K/1
  Add1/1 -> Divide1/2
  Constant1/1 -> Add1/2
  Gain3/1 -> Add1/1
  Add/1 -> Divide1/1, Cp/1
  Constant/1 -> Add/2
  Gain2/1 -> Add/1
  T1/1 -> Add2/1
  Tk/1 -> Add2/2
  Add2/1 -> Gain2/1, Gain3/1

== system ranqilunji/PT/turbine_TN/K1 ==
  note: Cp
  note: Cv
  T1 : Inport
  Add : Sum
  Add1 : Sum
  Add2 : Sum  Inputs=+-
  Constant : Constant  Value=0.9956
  Constant1 : Constant  Value=0.7088
  Divide1 : Product  Inputs=*/
  Gain2 : Gain  Gain=0.000093
  Gain3 : Gain  Gain=0.000093
  Tk : Constant  Value=273.15
  K : Outport
  Cp : Outport  Port=2
  wires:
  Add/1 -> Divide1/1, Cp/1
  Constant/1 -> Add/2
  Gain2/1 -> Add/1
  T1/1 -> Add2/1
  Tk/1 -> Add2/2
  Add2/1 -> Gain2/1, Gain3/1
  Divide1/1 -> K/1
  Add1/1 -> Divide1/2
  Constant1/1 -> Add1/2
  Gain3/1 -> Add1/1
